simulink model "MVS_Dynamic_Trigger_Two_Layers_NoRA"  (R2024a)
settings: Solver=ode5  StartTime=0.0  StopTime=180  FixedStep=0.01  RelTol=1e-3
(part 3 of 4)

== matlab function MVS_Dynamic_Trigger_Two_Layers_NoRA/High-Level Agent 4/Information receiver ==
  data: e_tilde_xi output; info_indi input; info_all input; e_tilde_vi output; delta_xi output; delta_vi output; acl_ref_agent output; Laplacian input
function [e_tilde_xi, e_tilde_vi, delta_xi, delta_vi, acl_ref_agent] = info_selector(info_indi, info_all, Laplacian)

%% Notation
% info_indi = [delta_xi, delta_vi, v_d_dot]
% info_all is the info obtained from event triggered communication, note
% that we cannot use this directly because each agent should know its own
% tracking errors
% Laplacian is the Laplacian matrix of the communication topology

%% Basic parameters
serial_num = 4;
dimension = 3;

%% Information selection
L_i = kron(Laplacian(serial_num, :), eye(3));
num_agent = size(Laplacian, 1);

% Current agent states
delta_xi = info_indi(1:3);
delta_vi = info_indi(4:6);
acl_ref_agent = info_indi(7:9);

% Select position error and the velocity error
delta_x_all = kron(eye(num_agent), [eye(dimension), zeros(dimension)]) * info_all;
delta_v_all = kron(eye(num_agent), [zeros(dimension), eye(dimension)]) * info_all;

% Replace the event-triggered error with its own real-time errors
delta_x_all( (serial_num - 1) * dimension + 1: serial_num * dimension ) = delta_xi;
delta_v_all( (serial_num - 1) * dimension + 1: serial_num * dimension ) = delta_vi;

% Calculate the cooperative errors
e_tilde_xi = L_i * delta_x_all;
e_tilde_vi = L_i * delta_v_all;

end

== matlab function MVS_Dynamic_Trigger_Two_Layers_NoRA/High-Level Agent 4/Trajectory Planner/Achievability assurance/Input compensator ==
  data: u_i_restrict input; v_i input; u_i_actual output; Xi_i input; Xi_i_dot output
function [u_i_actual, Xi_i_dot] = input_compensator(u_i_restrict, v_i, Xi_i)

%% Basic parameters
eta_1 = 10 * eye(3);
eta_2 = 0.5 * eye(3);
eta_3 = 6 * eye(3);
U_Mi = [2;2;1.5];

Xi_m = 5;

%% Preliminary compensation
v_Mi = [5;5;4];
control_step = 0.01;
v_up = v_Mi - v_i;
v_low = -v_Mi - v_i;
u_up = min(v_up/control_step, U_Mi);
u_low = max(v_low/control_step, -U_Mi);

%% Calculate the actual control input
u_i = u_i_restrict - eta_3 * Xi_i;
u_i_actual = u_i;

for i = 1 : size(u_i_actual,1)
    if u_i(i) > u_up(i)
        u_i_actual(i) = u_up(i);
    elseif u_i(i) < u_low(i)
        u_i_actual(i) = u_low(i);
    end
end

u_tilde_i = u_i - u_i_actual;

if norm(Xi_i) < Xi_m
    Xi_i_dot = eta_1 * u_tilde_i - eta_2 * Xi_i;
else
    Xi_i_dot = eta_1 * u_tilde_i - eta_2 * Xi_i - norm(u_tilde_i)^2/norm(Xi_i)^2;
end

end

== matlab function MVS_Dynamic_Trigger_Two_Layers_NoRA/High-Level Agent 4/Trajectory Planner/Achievability assurance/Nominal SMC ==
  data: delta_x input; u_restrict output; delta_v input; a_d input; delta_norm output
function [u_restrict, delta_norm] = slide_control(delta_x, delta_v, a_d)

c = 1 * eye(3);
lambda = 1 * eye(3);
r_1 = 1.5;        % Maximum difference
% r_2 = 0.5;
k_tilde = 2;

s = delta_v + lambda * delta_x;
delta_norm = norm(delta_x);

choice = 1;

switch choice
    case 1
        u_restrict = a_d - lambda * delta_v - c * s - k_tilde /(r_1^2 - norm(delta_x)^2) * delta_x;
    case 2
        u_restrict = a_d - lambda * delta_v - c * s - delta_x;
    case 3
        u_restrict = - lambda * delta_v - c * s - k_tilde * 3 * delta_x / (r_1^2 - norm(delta_x)^2);
    case 4
        u_restrict = - lambda * delta_v - c * s - k_tilde * delta_x;
end

%% Known physical acceleration
% u_restrict = a_d - lambda * delta_v - (r_1^2 - norm(s)^2) * c * s;
% u_restrict = a_d - lambda * delta_v - c * s - 2 * max(3 /(r_1^2 - norm(delta_x)^2), 1) * delta_x;
% u_restrict = a_d - lambda * delta_v - c * s - 2 * (r_1^2 - r_2^2) /(r_1^2 - norm(delta_x)^2) * delta_x;
% u_restrict = a_d - lambda * delta_v - c * s - delta_x;

%% Unknown physical acceleration
% u_restrict = - lambda * delta_v - c * s - 2 * 3 * delta_x / (r_1^2 - norm(delta_x)^2);
% u_restrict = - lambda * delta_v - c * s - 2 * delta_x;

end

== matlab function MVS_Dynamic_Trigger_Two_Layers_NoRA/High-Level Agent 4/Trajectory Planner/Cooperative tracking/Input compensator ==
  data: u_i_slide input; v_i input; u_i_actual output; Xi_i input; Xi_i_dot output
function [u_i_actual, Xi_i_dot] = input_compensator(u_i_slide, v_i, Xi_i)

%% Basic parameters
eta_1 = 10 * eye(3);
eta_2 = 0.5 * eye(3);
eta_3 = 6 * eye(3);
U_Mi = [2;2;1.5];

Xi_m = 5;

%% Preliminary compensation
v_Mi = [5;5;4];
control_step = 0.01;
v_up = v_Mi - v_i;
v_low = -v_Mi - v_i;
u_up = min(v_up/control_step, U_Mi);
u_low = max(v_low/control_step, -U_Mi);

%% Calculate the actual control input
u_i = u_i_slide - eta_3 * Xi_i;
u_i_actual = u_i;

for i = 1 : size(u_i_actual,1)
    if u_i(i) > u_up(i)
        u_i_actual(i) = u_up(i);
    elseif u_i(i) < u_low(i)
        u_i_actual(i) = u_low(i);
    end
end

u_tilde_i = u_i - u_i_actual;

if norm(Xi_i) < Xi_m
    Xi_i_dot = eta_1 * u_tilde_i - eta_2 * Xi_i;
else
    Xi_i_dot = eta_1 * u_tilde_i - eta_2 * Xi_i - norm(u_tilde_i)^2/norm(Xi_i)^2;
end

end

== matlab function MVS_Dynamic_Trigger_Two_Layers_NoRA/Communication Preparation 5/Event Tigger Mechanism/Event trigger ==
  data: time input; E_norm output; trigger_flag output; info_trigger output; delta_xi_now input; beta_i output; delta_vi_now input; e_tilde input; info_prev input; beta_i_prev input
function [E_norm, trigger_flag, info_trigger, beta_i] = event_trigger_commu(time, delta_xi_now, delta_vi_now, e_tilde, info_prev, beta_i_prev)

dimension = 3;

commu_step = 0.01;
step_size = 0.01;

if mod(time,commu_step) == 0

    E_xi = delta_xi_now - info_prev(dimension * 0 + 1 : dimension * 1);
    E_vi = delta_vi_now - info_prev(dimension * 1 + 1 : dimension * 2);
    trigger_flag = 0;
    info_trigger = info_prev;
    
    Q_max = 3.0;
    A_tilde = 2.5;
    P_min = 0.4;
    Lambda_min = 2;
    C_i = 2* eye(3);
    Lambda_i = 2* eye(3);
    rho_2 = 0.3;
    rho_3 = 0.5;
    alpha_1 = 1;
    
    gamma_2 = 0.5;
    
    F_2 = norm(Q_max * A_tilde * C_i * E_vi)^2/2 + norm(Q_max * A_tilde * C_i * Lambda_i * E_xi)^2/2 + 5 * rho_2 * P_min * Lambda_min * A_tilde^2 * norm(E_xi)^2 - 3 * rho_2 * P_min * Lambda_min * norm(e_tilde)^2/4;
    
    % Trigger check
    if F_2 - gamma_2 * beta_i_prev >=0
        trigger_flag = 1;
        F_2 = - 3 * rho_2 * P_min * Lambda_min * norm(e_tilde)^2/4;
        info_trigger = [delta_xi_now; delta_vi_now];
    end
    
    % If we abandon the event triggered scheme
    % info_trigger = [delta_xi_now; delta_vi_now];
    
    E_norm = norm(info_trigger - [delta_xi_now; delta_vi_now]);
    
    beta_i_dot = - alpha_1 * beta_i_prev - F_2 + rho_3;
    
    beta_i = beta_i_prev + beta_i_dot * step_size;

else
    info_trigger = info_prev;
    E_norm = norm(info_trigger - [delta_xi_now; delta_vi_now]);
    trigger_flag = 0;
    beta_i = beta_i_prev;
end

end

== matlab function MVS_Dynamic_Trigger_Two_Layers_NoRA/Communication Preparation 5/Reference Filter/Adaptive filter/Input compensator ==
  data: u_i_nom input; u_i output; Xi_i input; Xi_i_dot output
function [u_i, Xi_i_dot] = input_compensator(u_i_nom, Xi_i)

%% Basic parameters
eta_1 = 10 * eye(3);
eta_2 = 0.5 * eye(3);
eta_3 = 6 * eye(3);
v_Mi = [5;5;4];

Xi_m = 5;

%% Calculate the actual control input
u_i = u_i_nom - eta_3 * Xi_i;
u_i_actual = u_i;

u_up = v_Mi;
u_low = - v_Mi;

for i = 1 : size(u_i_actual,1)
    if u_i(i) > u_up(i)
        u_i_actual(i) = u_up(i);
    elseif u_i(i) < u_low(i)
        u_i_actual(i) = u_low(i);
    end
end

u_tilde_i = u_i - u_i_actual;

if norm(Xi_i) < Xi_m
    Xi_i_dot = eta_1 * u_tilde_i - eta_2 * Xi_i;
else
    Xi_i_dot = eta_1 * u_tilde_i - eta_2 * Xi_i - norm(u_tilde_i)^2/norm(Xi_i)^2;
end

% Xi_i_dot = [0;0;0];

end

== matlab function MVS_Dynamic_Trigger_Two_Layers_NoRA/High-Level Agent 5/Information receiver ==
  data: e_tilde_xi output; info_indi input; info_all input; e_tilde_vi output; delta_xi output; delta_vi output; acl_ref_agent output; Laplacian input
function [e_tilde_xi, e_tilde_vi, delta_xi, delta_vi, acl_ref_agent] = info_selector(info_indi, info_all, Laplacian)

%% Notation
% info_indi = [delta_xi, delta_vi, v_d_dot]
% info_all is the info obtained from event triggered communication, note
% that we cannot use this directly because each agent should know its own
% tracking errors
% Laplacian is the Laplacian matrix of the communication topology

%% Basic parameters
serial_num = 5;
dimension = 3;

%% Information selection
L_i = kron(Laplacian(serial_num, :), eye(3));
num_agent = size(Laplacian, 1);

% Current agent states
delta_xi = info_indi(1:3);
delta_vi = info_indi(4:6);
acl_ref_agent = info_indi(7:9);

% Select position error and the velocity error
delta_x_all = kron(eye(num_agent), [eye(dimension), zeros(dimension)]) * info_all;
delta_v_all = kron(eye(num_agent), [zeros(dimension), eye(dimension)]) * info_all;

% Replace the event-triggered error with its own real-time errors
delta_x_all( (serial_num - 1) * dimension + 1: serial_num * dimension ) = delta_xi;
delta_v_all( (serial_num - 1) * dimension + 1: serial_num * dimension ) = delta_vi;

% Calculate the cooperative errors
e_tilde_xi = L_i * delta_x_all;
e_tilde_vi = L_i * delta_v_all;

end

== matlab function MVS_Dynamic_Trigger_Two_Layers_NoRA/High-Level Agent 1/Information receiver ==
  data: e_tilde_xi output; info_indi input; info_all input; e_tilde_vi output; delta_xi output; delta_vi output; acl_ref_agent output; Laplacian input
function [e_tilde_xi, e_tilde_vi, delta_xi, delta_vi, acl_ref_agent] = info_selector(info_indi, info_all, Laplacian)

%% Notation
% info_indi = [delta_xi, delta_vi, v_d_dot]
% info_all is the info obtained from event triggered communication, note
% that we cannot use this directly because each agent should know its own
% tracking errors
% Laplacian is the Laplacian matrix of the communication topology

%% Basic parameters
serial_num = 1;
dimension = 3;

%% Information selection
L_i = kron(Laplacian(serial_num, :), eye(3));
num_agent = size(Laplacian, 1);

% Current agent states
delta_xi = info_indi(1:3);
delta_vi = info_indi(4:6);
acl_ref_agent = info_indi(7:9);

% Select position error and the velocity error
delta_x_all = kron(eye(num_agent), [eye(dimension), zeros(dimension)]) * info_all;
delta_v_all = kron(eye(num_agent), [zeros(dimension), eye(dimension)]) * info_all;

% Replace the event-triggered error with its own real-time errors
delta_x_all( (serial_num - 1) * dimension + 1: serial_num * dimension ) = delta_xi;
delta_v_all( (serial_num - 1) * dimension + 1: serial_num * dimension ) = delta_vi;

% Calculate the cooperative errors
e_tilde_xi = L_i * delta_x_all;
e_tilde_vi = L_i * delta_v_all;

end

== matlab function MVS_Dynamic_Trigger_Two_Layers_NoRA/High-Level Agent 5/Trajectory Planner/Achievability assurance/Input compensator ==
  data: u_i_restrict input; v_i input; u_i_actual output; Xi_i input; Xi_i_dot output
function [u_i_actual, Xi_i_dot] = input_compensator(u_i_restrict, v_i, Xi_i)

%% Basic parameters
eta_1 = 10 * eye(3);
eta_2 = 0.5 * eye(3);
eta_3 = 6 * eye(3);
U_Mi = [2;2;1.5];

Xi_m = 5;

%% Preliminary compensation
v_Mi = [5;5;4];
control_step = 0.01;
v_up = v_Mi - v_i;
v_low = -v_Mi - v_i;
u_up = min(v_up/control_step, U_Mi);
u_low = max(v_low/control_step, -U_Mi);

%% Calculate the actual control input
u_i = u_i_restrict - eta_3 * Xi_i;
u_i_actual = u_i;

for i = 1 : size(u_i_actual,1)
    if u_i(i) > u_up(i)
        u_i_actual(i) = u_up(i);
    elseif u_i(i) < u_low(i)
        u_i_actual(i) = u_low(i);
    end
end

u_tilde_i = u_i - u_i_actual;

if norm(Xi_i) < Xi_m
    Xi_i_dot = eta_1 * u_tilde_i - eta_2 * Xi_i;
else
    Xi_i_dot = eta_1 * u_tilde_i - eta_2 * Xi_i - norm(u_tilde_i)^2/norm(Xi_i)^2;
end

end

== matlab function MVS_Dynamic_Trigger_Two_Layers_NoRA/High-Level Agent 5/Trajectory Planner/Achievability assurance/Nominal SMC ==
  data: delta_x input; u_restrict output; delta_v input; a_d input; delta_norm output
function [u_restrict, delta_norm] = slide_control(delta_x, delta_v, a_d)

c = 1 * eye(3);
lambda = 1 * eye(3);
r_1 = 1.5;        % Maximum difference
% r_2 = 0.5;
k_tilde = 2;

s = delta_v + lambda * delta_x;
delta_norm = norm(delta_x);

choice = 1;

switch choice
    case 1
        u_restrict = a_d - lambda * delta_v - c * s - k_tilde /(r_1^2 - norm(delta_x)^2) * delta_x;
    case 2
        u_restrict = a_d - lambda * delta_v - c * s - delta_x;
    case 3
        u_restrict = - lambda * delta_v - c * s - k_tilde * 3 * delta_x / (r_1^2 - norm(delta_x)^2);
    case 4
        u_restrict = - lambda * delta_v - c * s - k_tilde * delta_x;
end

%% Known physical acceleration
% u_restrict = a_d - lambda * delta_v - (r_1^2 - norm(s)^2) * c * s;
% u_restrict = a_d - lambda * delta_v - c * s - 2 * max(3 /(r_1^2 - norm(delta_x)^2), 1) * delta_x;
% u_restrict = a_d - lambda * delta_v - c * s - 2 * (r_1^2 - r_2^2) /(r_1^2 - norm(delta_x)^2) * delta_x;
% u_restrict = a_d - lambda * delta_v - c * s - delta_x;

%% Unknown physical acceleration
% u_restrict = - lambda * delta_v - c * s - 2 * 3 * delta_x / (r_1^2 - norm(delta_x)^2);
% u_restrict = - lambda * delta_v - c * s - 2 * delta_x;

end

== matlab function MVS_Dynamic_Trigger_Two_Layers_NoRA/High-Level Agent 5/Trajectory Planner/Cooperative tracking/Input compensator ==
  data: u_i_slide input; v_i input; u_i_actual output; Xi_i input; Xi_i_dot output
function [u_i_actual, Xi_i_dot] = input_compensator(u_i_slide, v_i, Xi_i)

%% Basic parameters
eta_1 = 10 * eye(3);
eta_2 = 0.5 * eye(3);
eta_3 = 6 * eye(3);
U_Mi = [2;2;1.5];

Xi_m = 5;

%% Preliminary compensation
v_Mi = [5;5;4];
control_step = 0.01;
v_up = v_Mi - v_i;
v_low = -v_Mi - v_i;
u_up = min(v_up/control_step, U_Mi);
u_low = max(v_low/control_step, -U_Mi);

%% Calculate the actual control input
u_i = u_i_slide - eta_3 * Xi_i;
u_i_actual = u_i;

for i = 1 : size(u_i_actual,1)
    if u_i(i) > u_up(i)
        u_i_actual(i) = u_up(i);
    elseif u_i(i) < u_low(i)
        u_i_actual(i) = u_low(i);
    end
end

u_tilde_i = u_i - u_i_actual;

if norm(Xi_i) < Xi_m
    Xi_i_dot = eta_1 * u_tilde_i - eta_2 * Xi_i;
else
    Xi_i_dot = eta_1 * u_tilde_i - eta_2 * Xi_i - norm(u_tilde_i)^2/norm(Xi_i)^2;
end

end

== matlab function MVS_Dynamic_Trigger_Two_Layers_NoRA/Communication Preparation 6/Event Tigger Mechanism/Event trigger ==
  data: time input; E_norm output; trigger_flag output; info_trigger output; delta_xi_now input; beta_i output; delta_vi_now input; e_tilde input; info_prev input; beta_i_prev input
function [E_norm, trigger_flag, info_trigger, beta_i] = event_trigger_commu(time, delta_xi_now, delta_vi_now, e_tilde, info_prev, beta_i_prev)

dimension = 3;

commu_step = 0.01;
step_size = 0.01;

if mod(time,commu_step) == 0

    E_xi = delta_xi_now - info_prev(dimension * 0 + 1 : dimension * 1);
    E_vi = delta_vi_now - info_prev(dimension * 1 + 1 : dimension * 2);
    trigger_flag = 0;
    info_trigger = info_prev;
    
    Q_max = 3.0;
    A_tilde = 2.5;
    P_min = 0.4;
    Lambda_min = 2;
    C_i = 2* eye(3);
    Lambda_i = 2* eye(3);
    rho_2 = 0.3;
    rho_3 = 0.5;
    alpha_1 = 1;
    
    gamma_2 = 0.5;
    
    F_2 = norm(Q_max * A_tilde * C_i * E_vi)^2/2 + norm(Q_max * A_tilde * C_i * Lambda_i * E_xi)^2/2 + 5 * rho_2 * P_min * Lambda_min * A_tilde^2 * norm(E_xi)^2 - 3 * rho_2 * P_min * Lambda_min * norm(e_tilde)^2/4;
    
    % Trigger check
    if F_2 - gamma_2 * beta_i_prev >=0
        trigger_flag = 1;
        F_2 = - 3 * rho_2 * P_min * Lambda_min * norm(e_tilde)^2/4;
        info_trigger = [delta_xi_now; delta_vi_now];
    end
    
    % If we abandon the event triggered scheme
    % info_trigger = [delta_xi_now; delta_vi_now];
    
    E_norm = norm(info_trigger - [delta_xi_now; delta_vi_now]);
    
    beta_i_dot = - alpha_1 * beta_i_prev - F_2 + rho_3;
    
    beta_i = beta_i_prev + beta_i_dot * step_size;

else
    info_trigger = info_prev;
    E_norm = norm(info_trigger - [delta_xi_now; delta_vi_now]);
    trigger_flag = 0;
    beta_i = beta_i_prev;
end

end

== matlab function MVS_Dynamic_Trigger_Two_Layers_NoRA/Communication Preparation 6/Reference Filter/Adaptive filter/Input compensator ==
  data: u_i_nom input; u_i output; Xi_i input; Xi_i_dot output
function [u_i, Xi_i_dot] = input_compensator(u_i_nom, Xi_i)

%% Basic parameters
eta_1 = 10 * eye(3);
eta_2 = 0.5 * eye(3);
eta_3 = 6 * eye(3);
v_Mi = [5;5;4];

Xi_m = 5;

%% Calculate the actual control input
u_i = u_i_nom - eta_3 * Xi_i;
u_i_actual = u_i;

u_up = v_Mi;
u_low = - v_Mi;

for i = 1 : size(u_i_actual,1)
    if u_i(i) > u_up(i)
        u_i_actual(i) = u_up(i);
    elseif u_i(i) < u_low(i)
        u_i_actual(i) = u_low(i);
    end
end

u_tilde_i = u_i - u_i_actual;

if norm(Xi_i) < Xi_m
    Xi_i_dot = eta_1 * u_tilde_i - eta_2 * Xi_i;
else
    Xi_i_dot = eta_1 * u_tilde_i - eta_2 * Xi_i - norm(u_tilde_i)^2/norm(Xi_i)^2;
end

% Xi_i_dot = [0;0;0];

end

== matlab function MVS_Dynamic_Trigger_Two_Layers_NoRA/High-Level Agent 6/Information receiver ==
  data: e_tilde_xi output; info_indi input; info_all input; e_tilde_vi output; delta_xi output; delta_vi output; acl_ref_agent output; Laplacian input
function [e_tilde_xi, e_tilde_vi, delta_xi, delta_vi, acl_ref_agent] = info_selector(info_indi, info_all, Laplacian)

%% Notation
% info_indi = [delta_xi, delta_vi, v_d_dot]
% info_all is the info obtained from event triggered communication, note
% that we cannot use this directly because each agent should know its own
% tracking errors
% Laplacian is the Laplacian matrix of the communication topology

%% Basic parameters
serial_num = 6;
dimension = 3;

%% Information selection
L_i = kron(Laplacian(serial_num, :), eye(3));
num_agent = size(Laplacian, 1);

% Current agent states
delta_xi = info_indi(1:3);
delta_vi = info_indi(4:6);
acl_ref_agent = info_indi(7:9);

% Select position error and the velocity error
delta_x_all = kron(eye(num_agent), [eye(dimension), zeros(dimension)]) * info_all;
delta_v_all = kron(eye(num_agent), [zeros(dimension), eye(dimension)]) * info_all;

% Replace the event-triggered error with its own real-time errors
delta_x_all( (serial_num - 1) * dimension + 1: serial_num * dimension ) = delta_xi;
delta_v_all( (serial_num - 1) * dimension + 1: serial_num * dimension ) = delta_vi;

% Calculate the cooperative errors
e_tilde_xi = L_i * delta_x_all;
e_tilde_vi = L_i * delta_v_all;

end

== matlab function MVS_Dynamic_Trigger_Two_Layers_NoRA/High-Level Agent 6/Trajectory Planner/Achievability assurance/Input compensator ==
  data: u_i_restrict input; v_i input; u_i_actual output; Xi_i input; Xi_i_dot output
function [u_i_actual, Xi_i_dot] = input_compensator(u_i_restrict, v_i, Xi_i)

%% Basic parameters
eta_1 = 10 * eye(3);
eta_2 = 0.5 * eye(3);
eta_3 = 6 * eye(3);
U_Mi = [2;2;1.5];

Xi_m = 5;

%% Preliminary compensation
v_Mi = [5;5;4];
control_step = 0.01;
v_up = v_Mi - v_i;
v_low = -v_Mi - v_i;
u_up = min(v_up/control_step, U_Mi);
u_low = max(v_low/control_step, -U_Mi);

%% Calculate the actual control input
u_i = u_i_restrict - eta_3 * Xi_i;
u_i_actual = u_i;

for i = 1 : size(u_i_actual,1)
    if u_i(i) > u_up(i)
        u_i_actual(i) = u_up(i);
    elseif u_i(i) < u_low(i)
        u_i_actual(i) = u_low(i);
    end
end

u_tilde_i = u_i - u_i_actual;

if norm(Xi_i) < Xi_m
    Xi_i_dot = eta_1 * u_tilde_i - eta_2 * Xi_i;
else
    Xi_i_dot = eta_1 * u_tilde_i - eta_2 * Xi_i - norm(u_tilde_i)^2/norm(Xi_i)^2;
end

end

== matlab function MVS_Dynamic_Trigger_Two_Layers_NoRA/High-Level Agent 6/Trajectory Planner/Achievability assurance/Nominal SMC ==
  data: delta_x input; u_restrict output; delta_v input; a_d input; delta_norm output
function [u_restrict, delta_norm] = slide_control(delta_x, delta_v, a_d)

c = 1 * eye(3);
lambda = 1 * eye(3);
r_1 = 1.5;        % Maximum difference
% r_2 = 0.5;
k_tilde = 2;

s = delta_v + lambda * delta_x;
delta_norm = norm(delta_x);

choice = 1;

switch choice
    case 1
        u_restrict = a_d - lambda * delta_v - c * s - k_tilde /(r_1^2 - norm(delta_x)^2) * delta_x;
    case 2
        u_restrict = a_d - lambda * delta_v - c * s - delta_x;
    case 3
        u_restrict = - lambda * delta_v - c * s - k_tilde * 3 * delta_x / (r_1^2 - norm(delta_x)^2);
    case 4
        u_restrict = - lambda * delta_v - c * s - k_tilde * delta_x;
end

%% Known physical acceleration
% u_restrict = a_d - lambda * delta_v - (r_1^2 - norm(s)^2) * c * s;
% u_restrict = a_d - lambda * delta_v - c * s - 2 * max(3 /(r_1^2 - norm(delta_x)^2), 1) * delta_x;
% u_restrict = a_d - lambda * delta_v - c * s - 2 * (r_1^2 - r_2^2) /(r_1^2 - norm(delta_x)^2) * delta_x;
% u_restrict = a_d - lambda * delta_v - c * s - delta_x;

%% Unknown physical acceleration
% u_restrict = - lambda * delta_v - c * s - 2 * 3 * delta_x / (r_1^2 - norm(delta_x)^2);
% u_restrict = - lambda * delta_v - c * s - 2 * delta_x;

end

== matlab function MVS_Dynamic_Trigger_Two_Layers_NoRA/High-Level Agent 6/Trajectory Planner/Cooperative tracking/Input compensator ==
  data: u_i_slide input; v_i input; u_i_actual output; Xi_i input; Xi_i_dot output
function [u_i_actual, Xi_i_dot] = input_compensator(u_i_slide, v_i, Xi_i)

%% Basic parameters
eta_1 = 10 * eye(3);
eta_2 = 0.5 * eye(3);
eta_3 = 6 * eye(3);
U_Mi = [2;2;1.5];

Xi_m = 5;

%% Preliminary compensation
v_Mi = [5;5;4];
control_step = 0.01;
v_up = v_Mi - v_i;
v_low = -v_Mi - v_i;
u_up = min(v_up/control_step, U_Mi);
u_low = max(v_low/control_step, -U_Mi);

%% Calculate the actual control input
u_i = u_i_slide - eta_3 * Xi_i;
u_i_actual = u_i;

for i = 1 : size(u_i_actual,1)
    if u_i(i) > u_up(i)
        u_i_actual(i) = u_up(i);
    elseif u_i(i) < u_low(i)
        u_i_actual(i) = u_low(i);
    end
end

u_tilde_i = u_i - u_i_actual;

if norm(Xi_i) < Xi_m
    Xi_i_dot = eta_1 * u_tilde_i - eta_2 * Xi_i;
else
    Xi_i_dot = eta_1 * u_tilde_i - eta_2 * Xi_i - norm(u_tilde_i)^2/norm(Xi_i)^2;
end

end

== matlab function MVS_Dynamic_Trigger_Two_Layers_NoRA/Communication Preparation 1/Reference Filter/Adaptive filter/Input compensator ==
  data: u_i_nom input; u_i output; Xi_i input; Xi_i_dot output
function [u_i, Xi_i_dot] = input_compensator(u_i_nom, Xi_i)

%% Basic parameters
eta_1 = 10 * eye(3);
eta_2 = 0.5 * eye(3);
eta_3 = 6 * eye(3);
v_Mi = [5;5;4];

Xi_m = 5;

%% Calculate the actual control input
u_i = u_i_nom - eta_3 * Xi_i;
u_i_actual = u_i;

u_up = v_Mi;
u_low = - v_Mi;

for i = 1 : size(u_i_actual,1)
    if u_i(i) > u_up(i)
        u_i_actual(i) = u_up(i);
    elseif u_i(i) < u_low(i)
        u_i_actual(i) = u_low(i);
    end
end

u_tilde_i = u_i - u_i_actual;

if norm(Xi_i) < Xi_m
    Xi_i_dot = eta_1 * u_tilde_i - eta_2 * Xi_i;
else
    Xi_i_dot = eta_1 * u_tilde_i - eta_2 * Xi_i - norm(u_tilde_i)^2/norm(Xi_i)^2;
end

% Xi_i_dot = [0;0;0];

end

== matlab function MVS_Dynamic_Trigger_Two_Layers_NoRA/Communication Preparation 1/Reference Filter/Adaptive filter/Nominal filter ==
  data: pos_ref input; u_i_nom output; vel_ref input; current_pos input; filter_error output
function [u_i_nom, filter_error]= nominal_filter(pos_ref, vel_ref, current_pos)

filter_error = current_pos - pos_ref;
k = 2 * eye(3);

u_i_nom = - k * filter_error + vel_ref;

end

== matlab function MVS_Dynamic_Trigger_Two_Layers_NoRA/Overall reference/Ref_gene ==
  data: t input; pos_ref output; vel_ref output; acc_ref output
function [pos_ref, vel_ref, acc_ref] = position_ref(t)

%% The first 4 vehicles are ground vehicles, while the rest are aerial vehicles
%% The reference contains three stages
t_1 = 30;
t_2 = 90;

if t < t_1
    %% Stage 1: Use linear references, simulate the scenario of assemble
    x_initial = -30;
    y_initial = -25;
    x_vel = 3;
    y_vel = 1.5;
    x_distance = 8;
    y_distance = 4;

    x_1 = [x_initial + x_vel * t - x_distance * 0; y_initial + y_vel * t - y_distance * 0; 0];
    x_2 = [x_initial + x_vel * t - x_distance * 1; y_initial + y_vel * t - y_distance * 1; 0];
    x_3 = [x_initial + x_vel * t - x_distance * 2; y_initial + y_vel * t - y_distance * 2; 0];
    x_4 = [x_initial + x_vel * t - x_distance * 3; y_initial + y_vel * t - y_distance * 3; 0];
    x_5 = [x_initial + x_vel * t - x_distance * 1; y_initial + y_vel * t - y_distance * 1; 60];
    x_6 = [x_initial + x_vel * t - x_distance * 3; y_initial + y_vel * t - y_distance * 3; 60];

    v_1 = [x_vel; y_vel; 0];
    v_2 = [x_vel; y_vel; 0];
    v_3 = [x_vel; y_vel; 0];
    v_4 = [x_vel; y_vel; 0];
    v_5 = [x_vel; y_vel; 0];
    v_6 = [x_vel; y_vel; 0];

    a_1 = zeros(3,1);
    a_2 = zeros(3,1);
    a_3 = zeros(3,1);
    a_4 = zeros(3,1);
    a_5 = zeros(3,1);
    a_6 = zeros(3,1);

elseif t >= t_1 && t < t_2
    %% Stage 2: Use linear trajectories as reference, simulate straight roads
    x_initial = 65;
    y_initial = 25;
    x_vel = 3;
    y_vel = 3;
    x_distance = 8;
    y_distance = 6;

    x_1 = [x_initial + x_vel * (t - t_1) - x_distance * 0; y_initial + y_vel * (t - t_1) - y_distance * 0; 0];
    x_2 = [x_initial + x_vel * (t - t_1) - x_distance * 1; y_initial + y_vel * (t - t_1) - y_distance * 1; 0];
    x_3 = [x_initial + x_vel * (t - t_1) - x_distance * 2; y_initial + y_vel * (t - t_1) - y_distance * 2; 0];
    x_4 = [x_initial + x_vel * (t - t_1) - x_distance * 3; y_initial + y_vel * (t - t_1) - y_distance * 3; 0];
    x_5 = [x_initial + x_vel * (t - t_1) - x_distance * 1; y_initial + y_vel * (t - t_1) - y_distance * 1; 100];
    x_6 = [x_initial + x_vel * (t - t_1) - x_distance * 3; y_initial + y_vel * (t - t_1) - y_distance * 3; 100];

    v_1 = [x_vel; y_vel; 0];
    v_2 = [x_vel; y_vel; 0];
    v_3 = [x_vel; y_vel; 0];
    v_4 = [x_vel; y_vel; 0];
    v_5 = [x_vel; y_vel; 0];
    v_6 = [x_vel; y_vel; 0];

    a_1 = zeros(3,1);
    a_2 = zeros(3,1);
    a_3 = zeros(3,1);
    a_4 = zeros(3,1);
    a_5 = zeros(3,1);
    a_6 = zeros(3,1);

else
    %% Stage 3: Use nonlinear trajectories as reference, simulate complex roads
    x_initial = 245;
    y_initial = 205;
    x_vel = 3;
    y_vel = 0;
    curve_amp = 30;
    curve_ang_vel = 0.1;
    time_delay = 4;

    x_1 = [x_initial + x_vel * (t - t_2 - time_delay * 0); y_initial + curve_amp * sin(curve_ang_vel*(t - t_2 - time_delay * 0))+ y_vel * (t - t_2 - time_delay * 0); 0];
    x_2 = [x_initial + x_vel * (t - t_2 - time_delay * 1); y_initial + curve_amp * sin(curve_ang_vel*(t - t_2 - time_delay * 1))+ y_vel * (t - t_2 - time_delay * 1); 0];
    x_3 = [x_initial + x_vel * (t - t_2 - time_delay * 2); y_initial + curve_amp * sin(curve_ang_vel*(t - t_2 - time_delay * 2))+ y_vel * (t - t_2 - time_delay * 2); 0];
    x_4 = [x_initial + x_vel * (t - t_2 - time_delay * 3); y_initial + curve_amp * sin(curve_ang_vel*(t - t_2 - time_delay * 3))+ y_vel * (t - t_2 - time_delay * 3); 0];
    x_5 = [x_initial + x_vel * (t - t_2 - time_delay * 0); y_initial + curve_amp * sin(curve_ang_vel*(t - t_2 - time_delay * 0))+ y_vel * (t - t_2 - time_delay * 0); 100];
    x_6 = [x_initial + x_vel * (t - t_2 - time_delay * 2); y_initial + curve_amp * sin(curve_ang_vel*(t - t_2 - time_delay * 2))+ y_vel * (t - t_2 - time_delay * 2); 100];

    v_1 = [x_vel; y_vel + curve_amp * curve_ang_vel * cos(curve_ang_vel*(t - t_2 - time_delay * 0)); 0];
    v_2 = [x_vel; y_vel + curve_amp * curve_ang_vel * cos(curve_ang_vel*(t - t_2 - time_delay * 1)); 0];
    v_3 = [x_vel; y_vel + curve_amp * curve_ang_vel * cos(curve_ang_vel*(t - t_2 - time_delay * 2)); 0];
    v_4 = [x_vel; y_vel + curve_amp * curve_ang_vel * cos(curve_ang_vel*(t - t_2 - time_delay * 3)); 0];
    v_5 = [x_vel; y_vel + curve_amp * curve_ang_vel * cos(curve_ang_vel*(t - t_2 - time_delay * 0)); 0];
    v_6 = [x_vel; y_vel + curve_amp * curve_ang_vel * cos(curve_ang_vel*(t - t_2 - time_delay * 2)); 0];

    a_1 = [0; - curve_amp * curve_ang_vel^2 * sin(curve_ang_vel*(t - t_2 - time_delay * 0)); 0];
    a_2 = [0; - curve_amp * curve_ang_vel^2 * sin(curve_ang_vel*(t - t_2 - time_delay * 1)); 0];
    a_3 = [0; - curve_amp * curve_ang_vel^2 * sin(curve_ang_vel*(t - t_2 - time_delay * 2)); 0];
    a_4 = [0; - curve_amp * curve_ang_vel^2 * sin(curve_ang_vel*(t - t_2 - time_delay * 3)); 0];
    a_5 = [0; - curve_amp * curve_ang_vel^2 * sin(curve_ang_vel*(t - t_2 - time_delay * 0)); 0];
    a_6 = [0; - curve_amp * curve_ang_vel^2 * sin(curve_ang_vel*(t - t_2 - time_delay * 2)); 0];

end

pos_ref = [x_1; x_2; x_3; x_4; x_5; x_6];

vel_ref = [v_1; v_2; v_3; v_4; v_5; v_6];

acc_ref = [a_1; a_2; a_3; a_4; a_5; a_6];

end

== matlab function MVS_Dynamic_Trigger_Two_Layers_NoRA/High-Level Agent 2/Information receiver ==
  data: e_tilde_xi output; info_indi input; info_all input; e_tilde_vi output; delta_xi output; delta_vi output; acl_ref_agent output; Laplacian input
function [e_tilde_xi, e_tilde_vi, delta_xi, delta_vi, acl_ref_agent] = info_selector(info_indi, info_all, Laplacian)

%% Notation
% info_indi = [delta_xi, delta_vi, v_d_dot]
% info_all is the info obtained from event triggered communication, note
% that we cannot use this directly because each agent should know its own
% tracking errors
% Laplacian is the Laplacian matrix of the communication topology

%% Basic parameters
serial_num = 2;
dimension = 3;

%% Information selection
L_i = kron(Laplacian(serial_num, :), eye(3));
num_agent = size(Laplacian, 1);

% Current agent states
delta_xi = info_indi(1:3);
delta_vi = info_indi(4:6);
acl_ref_agent = info_indi(7:9);

% Select position error and the velocity error
delta_x_all = kron(eye(num_agent), [eye(dimension), zeros(dimension)]) * info_all;
delta_v_all = kron(eye(num_agent), [zeros(dimension), eye(dimension)]) * info_all;

% Replace the event-triggered error with its own real-time errors
delta_x_all( (serial_num - 1) * dimension + 1: serial_num * dimension ) = delta_xi;
delta_v_all( (serial_num - 1) * dimension + 1: serial_num * dimension ) = delta_vi;

% Calculate the cooperative errors
e_tilde_xi = L_i * delta_x_all;
e_tilde_vi = L_i * delta_v_all;

end

== matlab function MVS_Dynamic_Trigger_Two_Layers_NoRA/Communication Preparation 1/Reference Filter/Communication-Receiver ==
  data: ref_all input; pos_ref_agent output; vel_ref_agent output; acl_ref_agent output
function [pos_ref_agent, vel_ref_agent, acl_ref_agent] = info_selector(ref_all)

%% Basic parameters
serial_num = 1;
dimension = 3;
agent_num = 6;

%% Information selection
pos_ref_agent = ref_all(dimension * (serial_num - 1) + 1 : serial_num * dimension);
vel_ref_agent = ref_all(dimension * (serial_num - 1) + dimension * agent_num + 1 : serial_num * dimension + dimension * agent_num);
acl_ref_agent = ref_all(dimension * (serial_num - 1) + dimension * agent_num * 2 + 1 : serial_num * dimension + dimension * agent_num * 2);

end

== matlab function MVS_Dynamic_Trigger_Two_Layers_NoRA/Communication Preparation 1/Reference Filter/Error Calculation ==
  data: vel_cur input; pos_cur input; delta_xi output; delta_vi output; states_high input; filter_error input; high_error output
function [delta_xi, delta_vi, high_error]= error_cal(vel_cur, pos_cur, states_high, filter_error)

delta_xi = states_high(1:3) - pos_cur;
delta_vi = states_high(4:6) - vel_cur;
high_error = filter_error + delta_xi;

end

== matlab function MVS_Dynamic_Trigger_Two_Layers_NoRA/Communication Preparation 2/Reference Filter/Communication-Receiver ==
  data: ref_all input; pos_ref_agent output; vel_ref_agent output; acl_ref_agent output
function [pos_ref_agent, vel_ref_agent, acl_ref_agent] = info_selector(ref_all)

%% Basic parameters
serial_num = 2;
dimension = 3;
agent_num = 6;

%% Information selection
pos_ref_agent = ref_all(dimension * (serial_num - 1) + 1 : serial_num * dimension);
vel_ref_agent = ref_all(dimension * (serial_num - 1) + dimension * agent_num + 1 : serial_num * dimension + dimension * agent_num);
acl_ref_agent = ref_all(dimension * (serial_num - 1) + dimension * agent_num * 2 + 1 : serial_num * dimension + dimension * agent_num * 2);

end

== matlab function MVS_Dynamic_Trigger_Two_Layers_NoRA/Communication Preparation 2/Reference Filter/Error Calculation ==
  data: vel_cur input; pos_cur input; delta_xi output; delta_vi output; states_high input; filter_error input; high_error output
function [delta_xi, delta_vi, high_error]= error_cal(vel_cur, pos_cur, states_high, filter_error)

delta_xi = states_high(1:3) - pos_cur;
delta_vi = states_high(4:6) - vel_cur;
high_error = filter_error + delta_xi;

end

== matlab function MVS_Dynamic_Trigger_Two_Layers_NoRA/Communication Preparation 3/Reference Filter/Adaptive filter/Nominal filter ==
  data: pos_ref input; u_i_nom output; vel_ref input; current_pos input; filter_error output
function [u_i_nom, filter_error]= nominal_filter(pos_ref, vel_ref, current_pos)

filter_error = current_pos - pos_ref;
k = 2 * eye(3);

u_i_nom = - k * filter_error + vel_ref;

end

== matlab function MVS_Dynamic_Trigger_Two_Layers_NoRA/Communication Preparation 3/Reference Filter/Communication-Receiver ==
  data: ref_all input; pos_ref_agent output; vel_ref_agent output; acl_ref_agent output
function [pos_ref_agent, vel_ref_agent, acl_ref_agent] = info_selector(ref_all)

%% Basic parameters
serial_num = 3;
dimension = 3;
agent_num = 6;

%% Information selection
pos_ref_agent = ref_all(dimension * (serial_num - 1) + 1 : serial_num * dimension);
vel_ref_agent = ref_all(dimension * (serial_num - 1) + dimension * agent_num + 1 : serial_num * dimension + dimension * agent_num);
acl_ref_agent = ref_all(dimension * (serial_num - 1) + dimension * agent_num * 2 + 1 : serial_num * dimension + dimension * agent_num * 2);

end

== matlab function MVS_Dynamic_Trigger_Two_Layers_NoRA/Communication Preparation 3/Reference Filter/Error Calculation ==
  data: vel_cur input; pos_cur input; delta_xi output; delta_vi output; states_high input; filter_error input; high_error output
function [delta_xi, delta_vi, high_error]= error_cal(vel_cur, pos_cur, states_high, filter_error)

delta_xi = states_high(1:3) - pos_cur;
delta_vi = states_high(4:6) - vel_cur;
high_error = filter_error + delta_xi;

end

== matlab function MVS_Dynamic_Trigger_Two_Layers_NoRA/Communication Preparation 4/Reference Filter/Adaptive filter/Nominal filter ==
  data: pos_ref input; u_i_nom output; vel_ref input; current_pos input; filter_error output
function [u_i_nom, filter_error]= nominal_filter(pos_ref, vel_ref, current_pos)

filter_error = current_pos - pos_ref;
k = 2 * eye(3);

u_i_nom = - k * filter_error + vel_ref;

end

== matlab function MVS_Dynamic_Trigger_Two_Layers_NoRA/Communication Preparation 4/Reference Filter/Communication-Receiver ==
  data: ref_all input; pos_ref_agent output; vel_ref_agent output; acl_ref_agent output
function [pos_ref_agent, vel_ref_agent, acl_ref_agent] = info_selector(ref_all)

%% Basic parameters
serial_num = 4;
dimension = 3;
agent_num = 6;

%% Information selection
pos_ref_agent = ref_all(dimension * (serial_num - 1) + 1 : serial_num * dimension);
vel_ref_agent = ref_all(dimension * (serial_num - 1) + dimension * agent_num + 1 : serial_num * dimension + dimension * agent_num);
acl_ref_agent = ref_all(dimension * (serial_num - 1) + dimension * agent_num * 2 + 1 : serial_num * dimension + dimension * agent_num * 2);

end

== matlab function MVS_Dynamic_Trigger_Two_Layers_NoRA/Communication Preparation 4/Reference Filter/Error Calculation ==
  data: vel_cur input; pos_cur input; delta_xi output; delta_vi output; states_high input; filter_error input; high_error output
function [delta_xi, delta_vi, high_error]= error_cal(vel_cur, pos_cur, states_high, filter_error)

delta_xi = states_high(1:3) - pos_cur;
delta_vi = states_high(4:6) - vel_cur;
high_error = filter_error + delta_xi;

end

== matlab function MVS_Dynamic_Trigger_Two_Layers_NoRA/Communication Preparation 5/Reference Filter/Adaptive filter/Nominal filter ==
  data: pos_ref input; u_i_nom output; vel_ref input; current_pos input; filter_error output
function [u_i_nom, filter_error]= nominal_filter(pos_ref, vel_ref, current_pos)

filter_error = current_pos - pos_ref;
k = 2 * eye(3);

u_i_nom = - k * filter_error + vel_ref;

end

== matlab function MVS_Dynamic_Trigger_Two_Layers_NoRA/Communication Preparation 5/Reference Filter/Communication-Receiver ==
  data: ref_all input; pos_ref_agent output; vel_ref_agent output; acl_ref_agent output
function [pos_ref_agent, vel_ref_agent, acl_ref_agent] = info_selector(ref_all)

%% Basic parameters
serial_num = 5;
dimension = 3;
agent_num = 6;

%% Information selection
pos_ref_agent = ref_all(dimension * (serial_num - 1) + 1 : serial_num * dimension);
vel_ref_agent = ref_all(dimension * (serial_num - 1) + dimension * agent_num + 1 : serial_num * dimension + dimension * agent_num);
acl_ref_agent = ref_all(dimension * (serial_num - 1) + dimension * agent_num * 2 + 1 : serial_num * dimension + dimension * agent_num * 2);

end

== matlab function MVS_Dynamic_Trigger_Two_Layers_NoRA/Communication Preparation 5/Reference Filter/Error Calculation ==
  data: vel_cur input; pos_cur input; delta_xi output; delta_vi output; states_high input; filter_error input; high_error output
function [delta_xi, delta_vi, high_error]= error_cal(vel_cur, pos_cur, states_high, filter_error)

delta_xi = states_high(1:3) - pos_cur;
delta_vi = states_high(4:6) - vel_cur;
high_error = filter_error + delta_xi;

end

== matlab function MVS_Dynamic_Trigger_Two_Layers_NoRA/High-Level Agent 2/Trajectory Planner/Achievability assurance/Input compensator ==
  data: u_i_restrict input; v_i input; u_i_actual output; Xi_i input; Xi_i_dot output
function [u_i_actual, Xi_i_dot] = input_compensator(u_i_restrict, v_i, Xi_i)

%% Basic parameters
eta_1 = 10 * eye(3);
eta_2 = 0.5 * eye(3);
eta_3 = 6 * eye(3);
U_Mi = [2;2;1.5];

Xi_m = 5;

%% Preliminary compensation
v_Mi = [5;5;4];
control_step = 0.01;
v_up = v_Mi - v_i;
v_low = -v_Mi - v_i;
u_up = min(v_up/control_step, U_Mi);
u_low = max(v_low/control_step, -U_Mi);

%% Calculate the actual control input
u_i = u_i_restrict - eta_3 * Xi_i;
u_i_actual = u_i;

for i = 1 : size(u_i_actual,1)
    if u_i(i) > u_up(i)
        u_i_actual(i) = u_up(i);
    elseif u_i(i) < u_low(i)
        u_i_actual(i) = u_low(i);
    end
end

u_tilde_i = u_i - u_i_actual;

if norm(Xi_i) < Xi_m
    Xi_i_dot = eta_1 * u_tilde_i - eta_2 * Xi_i;
else
    Xi_i_dot = eta_1 * u_tilde_i - eta_2 * Xi_i - norm(u_tilde_i)^2/norm(Xi_i)^2;
end

end

== matlab function MVS_Dynamic_Trigger_Two_Layers_NoRA/Communication Preparation 6/Reference Filter/Adaptive filter/Nominal filter ==
  data: pos_ref input; u_i_nom output; vel_ref input; current_pos input; filter_error output
function [u_i_nom, filter_error]= nominal_filter(pos_ref, vel_ref, current_pos)

filter_error = current_pos - pos_ref;
k = 2 * eye(3);

u_i_nom = - k * filter_error + vel_ref;

end

== matlab function MVS_Dynamic_Trigger_Two_Layers_NoRA/Communication Preparation 6/Reference Filter/Communication-Receiver ==
  data: ref_all input; pos_ref_agent output; vel_ref_agent output; acl_ref_agent output
function [pos_ref_agent, vel_ref_agent, acl_ref_agent] = info_selector(ref_all)

%% Basic parameters
serial_num = 6;
dimension = 3;
agent_num = 6;

%% Information selection
pos_ref_agent = ref_all(dimension * (serial_num - 1) + 1 : serial_num * dimension);
vel_ref_agent = ref_all(dimension * (serial_num - 1) + dimension * agent_num + 1 : serial_num * dimension + dimension * agent_num);
acl_ref_agent = ref_all(dimension * (serial_num - 1) + dimension * agent_num * 2 + 1 : serial_num * dimension + dimension * agent_num * 2);

end

== matlab function MVS_Dynamic_Trigger_Two_Layers_NoRA/Communication Preparation 6/Reference Filter/Error Calculation ==
  data: vel_cur input; pos_cur input; delta_xi output; delta_vi output; states_high input; filter_error input; high_error output
function [delta_xi, delta_vi, high_error]= error_cal(vel_cur, pos_cur, states_high, filter_error)

delta_xi = states_high(1:3) - pos_cur;
delta_vi = states_high(4:6) - vel_cur;
high_error = filter_error + delta_xi;

end

== matlab function MVS_Dynamic_Trigger_Two_Layers_NoRA/High-Level Agent 1/Trajectory Planner/Achievability assurance/Nominal SMC ==
  data: delta_x input; u_restrict output; delta_v input; a_d input; delta_norm output
function [u_restrict, delta_norm] = slide_control(delta_x, delta_v, a_d)

c = 1 * eye(3);
lambda = 1 * eye(3);
r_1 = 1.5;
% r_2 = 0.5;
k_tilde = 2;

s = delta_v + lambda * delta_x;
delta_norm = norm(delta_x);

choice = 1;

switch choice
    case 1
        u_restrict = a_d - lambda * delta_v - c * s - k_tilde /(r_1^2 - norm(delta_x)^2) * delta_x;
    case 2
        u_restrict = a_d - lambda * delta_v - c * s - delta_x;
    case 3
        u_restrict = - lambda * delta_v - c * s - k_tilde * 3 * delta_x / (r_1^2 - norm(delta_x)^2);
    case 4
        u_restrict = - lambda * delta_v - c * s - k_tilde * delta_x;
end

%% Known physical acceleration
% u_restrict = a_d - lambda * delta_v - (r_1^2 - norm(s)^2) * c * s;
% u_restrict = a_d - lambda * delta_v - c * s - 2 * max(3 /(r_1^2 - norm(delta_x)^2), 1) * delta_x;
% u_restrict = a_d - lambda * delta_v - c * s - 2 * (r_1^2 - r_2^2) /(r_1^2 - norm(delta_x)^2) * delta_x;
% u_restrict = a_d - lambda * delta_v - c * s - delta_x;

%% Unknown physical acceleration
% u_restrict = - lambda * delta_v - c * s - 2 * 3 * delta_x / (r_1^2 - norm(delta_x)^2);
% u_restrict = - lambda * delta_v - c * s - 2 * delta_x;

end

== matlab function MVS_Dynamic_Trigger_Two_Layers_NoRA/High-Level Agent 1/Trajectory Planner/Cooperative tracking/Input compensator ==
  data: u_i_slide input; v_i input; u_i_actual output; Xi_i input; Xi_i_dot output
function [u_i_actual, Xi_i_dot] = input_compensator(u_i_slide, v_i, Xi_i)

%% Basic parameters
eta_1 = 10 * eye(3);
eta_2 = 0.5 * eye(3);
eta_3 = 6 * eye(3);
U_Mi = [2;2;1.5];

Xi_m = 5;

%% Preliminary compensation
v_Mi = [5;5;4];
control_step = 0.01;
v_up = v_Mi - v_i;
v_low = -v_Mi - v_i;
u_up = min(v_up/control_step, U_Mi);
u_low = max(v_low/control_step, -U_Mi);

%% Calculate the actual control input
u_i = u_i_slide - eta_3 * Xi_i;
u_i_actual = u_i;

for i = 1 : size(u_i_actual,1)
    if u_i(i) > u_up(i)
        u_i_actual(i) = u_up(i);
    elseif u_i(i) < u_low(i)
        u_i_actual(i) = u_low(i);
    end
end

u_tilde_i = u_i - u_i_actual;

if norm(Xi_i) < Xi_m
    Xi_i_dot = eta_1 * u_tilde_i - eta_2 * Xi_i;
else
    Xi_i_dot = eta_1 * u_tilde_i - eta_2 * Xi_i - norm(u_tilde_i)^2/norm(Xi_i)^2;
end

end

== matlab function MVS_Dynamic_Trigger_Two_Layers_NoRA/High-Level Agent 1/Trajectory Planner/Cooperative tracking/Nominal sliding mode controller ==
  data: u_i_slide output; e_tilde_xi input; e_tilde_vi input; delta_xi input; delta_vi input; acl_ref_agent input
function u_i_slide = nominal_sliding_controller(e_tilde_xi, e_tilde_vi, delta_xi, delta_vi, acl_ref_agent)

%% This is the nominal sliding mode controller for precise reference tracking

%% Basic parameters
C_i = 2 * eye(3);
Lambda_i = 2 * eye(3);

%% Controller
% Control input
S_tilde_i = e_tilde_vi + Lambda_i * e_tilde_xi;

u_i_slide = - C_i * S_tilde_i - Lambda_i * delta_vi - delta_xi + acl_ref_agent;

end

== matlab function MVS_Dynamic_Trigger_Two_Layers_NoRA/High-Level Agent 1/Trajectory Planner/Input compensator ==
  data: u_i_track input; u_i_restrict input; u_i output; delta_low_norm input
function u_i  = input_compensator(u_i_track, u_i_restrict, delta_low_norm)

%% Basic parameters
r_2 = 0.5;
r_3 = 0.8;

%% Calculate the actual control input
scenario = 2;

switch scenario
    case 1
        if delta_low_norm < r_2
            u_i = u_i_track;
        elseif delta_low_norm >= r_2 && delta_low_norm < r_3
            u_i = (r_3 - delta_low_norm)/(r_3 - r_2) * u_i_track + (delta_low_norm - r_2)/(r_3 - r_2) * u_i_restrict;
        else
            u_i = u_i_restrict;
        end

    case 2
        u_i = u_i_track;
end

end

== matlab function MVS_Dynamic_Trigger_Two_Layers_NoRA/High-Level Agent 1/Trajectory Planner/State select ==
  data: states_high input; v_i output; states_low input; delta_x_tilde output; delta_v_tilde output; a_d output
function [v_i, delta_x_tilde, delta_v_tilde, a_d] = state_select(states_high, states_low)

delta_x_tilde = states_high(1:3) - states_low(1:3);
delta_v_tilde = states_high(4:6) - states_low(4:6);
a_d = states_low(7:9);
v_i = states_high(4:6);

end

== matlab function MVS_Dynamic_Trigger_Two_Layers_NoRA/High-Level Agent 2/Trajectory Planner/State select ==
  data: states_high input; v_i output; states_low input; delta_x_tilde output; delta_v_tilde output; a_d output
function [v_i, delta_x_tilde, delta_v_tilde, a_d] = state_select(states_high, states_low)

delta_x_tilde = states_high(1:3) - states_low(1:3);
delta_v_tilde = states_high(4:6) - states_low(4:6);
a_d = states_low(7:9);
v_i = states_high(4:6);

end

== matlab function MVS_Dynamic_Trigger_Two_Layers_NoRA/Communication Preparation 2/Reference Filter/Adaptive filter/Input compensator ==
  data: u_i_nom input; u_i output; Xi_i input; Xi_i_dot output
function [u_i, Xi_i_dot] = input_compensator(u_i_nom, Xi_i)

%% Basic parameters
eta_1 = 10 * eye(3);
eta_2 = 0.5 * eye(3);
eta_3 = 6 * eye(3);
v_Mi = [5;5;4];

Xi_m = 5;

%% Calculate the actual control input
u_i = u_i_nom - eta_3 * Xi_i;
u_i_actual = u_i;

u_up = v_Mi;
u_low = - v_Mi;

for i = 1 : size(u_i_actual,1)
    if u_i(i) > u_up(i)
        u_i_actual(i) = u_up(i);
    elseif u_i(i) < u_low(i)
        u_i_actual(i) = u_low(i);
    end
end

u_tilde_i = u_i - u_i_actual;

if norm(Xi_i) < Xi_m
    Xi_i_dot = eta_1 * u_tilde_i - eta_2 * Xi_i;
else
    Xi_i_dot = eta_1 * u_tilde_i - eta_2 * Xi_i - norm(u_tilde_i)^2/norm(Xi_i)^2;
end

% Xi_i_dot = [0;0;0];

end

== matlab function MVS_Dynamic_Trigger_Two_Layers_NoRA/High-Level Agent 3/Trajectory Planner/Cooperative tracking/Nominal sliding mode controller ==
  data: u_i_slide output; e_tilde_xi input; e_tilde_vi input; delta_xi input; delta_vi input; acl_ref_agent input
function u_i_slide = nominal_sliding_controller(e_tilde_xi, e_tilde_vi, delta_xi, delta_vi, acl_ref_agent)

%% This is the nominal sliding mode controller for precise reference tracking

%% Basic parameters
C_i = 2 * eye(3);
Lambda_i = 2 * eye(3);

%% Controller
% Control input
S_tilde_i = e_tilde_vi + Lambda_i * e_tilde_xi;

u_i_slide = - C_i * S_tilde_i - Lambda_i * delta_vi - delta_xi + acl_ref_agent;

end

== matlab function MVS_Dynamic_Trigger_Two_Layers_NoRA/High-Level Agent 3/Trajectory Planner/Input compensator ==
  data: u_i_track input; u_i_restrict input; u_i output; delta_low_norm input
function u_i  = input_compensator(u_i_track, u_i_restrict, delta_low_norm)

%% Basic parameters
r_2 = 0.5;
r_3 = 0.8;

%% Calculate the actual control input
scenario = 2;

switch scenario
    case 1
        if delta_low_norm < r_2
            u_i = u_i_track;
        elseif delta_low_norm >= r_2 && delta_low_norm < r_3
            u_i = (r_3 - delta_low_norm)/(r_3 - r_2) * u_i_track + (delta_low_norm - r_2)/(r_3 - r_2) * u_i_restrict;
        else
            u_i = u_i_restrict;
        end

    case 2
        u_i = u_i_track;
end

end

== matlab function MVS_Dynamic_Trigger_Two_Layers_NoRA/High-Level Agent 3/Trajectory Planner/State select ==
  data: states_high input; v_i output; states_low input; delta_x_tilde output; delta_v_tilde output; a_d output
function [v_i, delta_x_tilde, delta_v_tilde, a_d] = state_select(states_high, states_low)

delta_x_tilde = states_high(1:3) - states_low(1:3);
delta_v_tilde = states_high(4:6) - states_low(4:6);
a_d = states_low(7:9);
v_i = states_high(4:6);

end

== matlab function MVS_Dynamic_Trigger_Two_Layers_NoRA/High-Level Agent 4/Trajectory Planner/Cooperative tracking/Nominal sliding mode controller ==
  data: u_i_slide output; e_tilde_xi input; e_tilde_vi input; delta_xi input; delta_vi input; acl_ref_agent input
function u_i_slide = nominal_sliding_controller(e_tilde_xi, e_tilde_vi, delta_xi, delta_vi, acl_ref_agent)

%% This is the nominal sliding mode controller for precise reference tracking

%% Basic parameters
C_i = 2 * eye(3);
Lambda_i = 2 * eye(3);

%% Controller
% Control input
S_tilde_i = e_tilde_vi + Lambda_i * e_tilde_xi;

u_i_slide = - C_i * S_tilde_i - Lambda_i * delta_vi - delta_xi + acl_ref_agent;

end

== matlab function MVS_Dynamic_Trigger_Two_Layers_NoRA/High-Level Agent 4/Trajectory Planner/Input compensator ==
  data: u_i_track input; u_i_restrict input; u_i output; delta_low_norm input
function u_i  = input_compensator(u_i_track, u_i_restrict, delta_low_norm)

%% Basic parameters
r_2 = 0.5;
r_3 = 0.8;

%% Calculate the actual control input
scenario = 2;

switch scenario
    case 1
        if delta_low_norm < r_2
            u_i = u_i_track;
        elseif delta_low_norm >= r_2 && delta_low_norm < r_3
            u_i = (r_3 - delta_low_norm)/(r_3 - r_2) * u_i_track + (delta_low_norm - r_2)/(r_3 - r_2) * u_i_restrict;
        else
            u_i = u_i_restrict;
        end

    case 2
        u_i = u_i_track;
end

end

== matlab function MVS_Dynamic_Trigger_Two_Layers_NoRA/High-Level Agent 4/Trajectory Planner/State select ==
  data: states_high input; v_i output; states_low input; delta_x_tilde output; delta_v_tilde output; a_d output
function [v_i, delta_x_tilde, delta_v_tilde, a_d] = state_select(states_high, states_low)

delta_x_tilde = states_high(1:3) - states_low(1:3);
delta_v_tilde = states_high(4:6) - states_low(4:6);
a_d = states_low(7:9);
v_i = states_high(4:6);

end
